simulink model "SEIR_model"  (R2023a)
settings: Solver=VariableStepAuto  StartTime=0.0  StopTime=100  RelTol=1e-3
values from neighbouring files (symbols this model uses):
  b = 1.2    [parameters_covid.mat]
  g = 0.1    [parameters_covid.mat]
  lambda = 0.166666666667    [parameters_covid.mat]
  N = 7500000    [parameters_covid.mat]
settings Model: Creator=mluser  LastModifiedBy=mluser

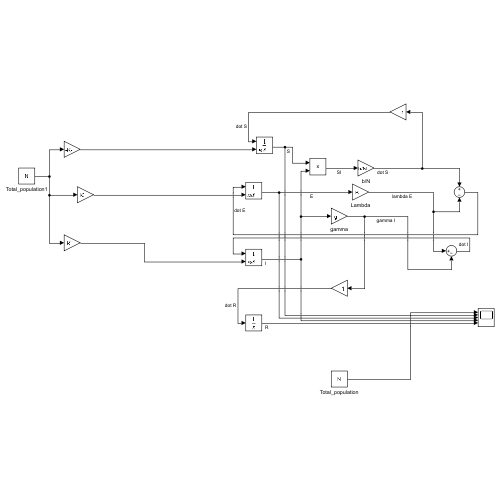
[thumbnail: Simulink's stored preview of the top-level diagram]
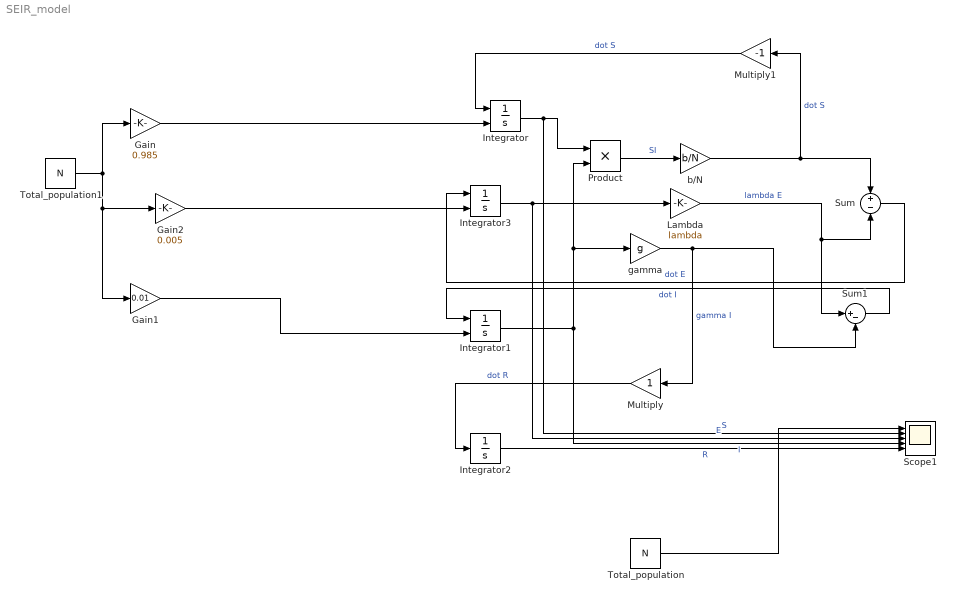
== system SEIR_model ==
  Gain : Gain  Gain=0.985
  Gain1 : Gain  Gain=0.01
  Gain2 : Gain  Gain=0.005
  Integrator : Integrator  InitialConditionSource=external  InitialCondition=N
  Integrator1 : Integrator  InitialConditionSource=external
  Integrator2 : Integrator
  Integrator3 : Integrator  InitialConditionSource=external
  Lambda : Gain  Gain=lambda
  Multiply : Gain
  Multiply1 : Gain  Gain=-1
  Product : Product
  Scope1 : Scope  NumInputPorts=5
  Sum : Sum  Inputs=+-
  Sum1 : Sum  Inputs=|+-
  Total_population : Constant  Value=N
  Total_population1 : Constant  Value=N
  b/N : Gain  Gain=b/N
  gamma : Gain  Gain=g
  wires:
  Integrator/1 -> Product/1, Scope1/2  "S"
  Product/1 -> b/N/1  "SI"
  gamma/1 -> Sum1/2, Multiply/1  "gamma I"
  Sum/1 -> Integrator3/1  "dot E"
  Multiply/1 -> Integrator2/1  "dot R"
  Integrator2/1 -> Scope1/5  "R"
  b/N/1 -> Multiply1/1, Sum/1  "dot S"
  Multiply1/1 -> Integrator/1  "dot S"
  Integrator1/1 -> gamma/1, Product/2, Scope1/4  "I"
  Gain/1 -> Integrator/2
  Gain1/1 -> Integrator1/2
  Total_population/1 -> Scope1/1
  Integrator3/1 -> Lambda/1, Scope1/3  "E"
  Total_population1/1 -> Gain1/1, Gain2/1, Gain/1
  Gain2/1 -> Integrator3/2
  Lambda/1 -> Sum/2, Sum1/1  "lambda E"
  Sum1/1 -> Integrator1/1  "dot I"
